simulink model "SpatialKineticsOffline"  (R2013a)
settings: Solver=ode4  StartTime=0.0  StopTime=tf  FixedStep=.001  RelTol=1e-3
PreLoadFcn:
  | load DarkLowerCoeffs
  | load DarkMiddleCoeffs
  | load DarkUpperCoeffs
  | load breaks
values from neighbouring files (symbols this model uses):
  alpha = [ -2.61*pcm -0.53*pcm ]    [SpatialKineticsOpenSourceMain.m]
  breaks = DarkLowerBreaks    [SpatialKineticsOpenSourceMain.m]
  BRIO = 4.266e7    (= 42660000)    [SpatialKineticsOpenSourceMain.m]
  cpc = 2414    [SpatialKineticsOpenSourceMain.m]
  cpp = 2414    [SpatialKineticsOpenSourceMain.m]
  DarkLowerCoeffs = ppDarkLower.coefs    [SpatialKineticsOpenSourceMain.m]
  DarkMiddleCoeffs = ppDarkMiddle.coefs    [SpatialKineticsOpenSourceMain.m]
  DarkRodWorthInserted = -5*Beta    (= -0.00815)    [SpatialKineticsOpenSourceMain.m]
  DarkUpperCoeffs = ppDarkUpper.coefs    [SpatialKineticsOpenSourceMain.m]
  downcomerTimeConstant = 5    [SpatialKineticsOpenSourceMain.m]
  downIO = 216.6*ones(1,3)    [SpatialKineticsOpenSourceMain.m]
  Kc1 = 1/(rho_secondary*V_secondary)    (= 0.00032726218348)    [SpatialKineticsOpenSourceMain.m]
  Kc2 = (h_secondary*A)/(cps*rho_secondary*V_secondary)    (= 1.23242359038)    [SpatialKineticsOpenSourceMain.m]
  Kh1 = 1/(rho_primary*V_primary)    (= 0.000447917898441)    [SpatialKineticsOpenSourceMain.m]
  Kh2 = (h_primary*A)/(cpp*rho_primary*V_primary)    (= 1.29038206968)    [SpatialKineticsOpenSourceMain.m]
  Kw1 = h_primary    (= 23800)    [SpatialKineticsOpenSourceMain.m]
  Kw2 = h_secondary    (= 24500)    [SpatialKineticsOpenSourceMain.m]
  Kw3 = A/(rho_tube*cpw*V_tube)    (= 0.000122049789882)    [SpatialKineticsOpenSourceMain.m]
  PHX_IO = [649.8 637.9 643.7]    [SpatialKineticsOpenSourceMain.m]
  PHX_PI_IO = 271.8    [SpatialKineticsOpenSourceMain.m]
  rate_pct = rate/100    [SpatialKineticsOfflineMain.m]
  rcp_activatetime = 20    [SpatialKineticsOpenSourceMain.m]
  rcpt = 0.1    [SpatialKineticsOpenSourceMain.m]
  reactor_PI_IO = 0.8574    [SpatialKineticsOpenSourceMain.m]
  SVIO = zeros(1,17)    [SpatialKineticsOpenSourceMain.m]
  Ts = 0.001    [SpatialKineticsOpenSourceMain.m]
  xfc0 = -Atemp\btemp*u0    [SpatialKineticsOpenSourceMain.m]
  zone1_IO = [1.041 0.01764 0.04848]    [SpatialKineticsOpenSourceMain.m]
  zone1_thermal_IO = [1044 658.3]    [SpatialKineticsOpenSourceMain.m]
  zone2_IO = [1.098 0.0186 0.05114]    [SpatialKineticsOpenSourceMain.m]
  zone2_thermal_IO = [1083 675.9]    [SpatialKineticsOpenSourceMain.m]
  zone3_IO = [0.9147 0.01549 0.04259]    [SpatialKineticsOpenSourceMain.m]
  zone3_thermal_IO = [1031 692.5]    [SpatialKineticsOpenSourceMain.m]
libraries: simulink x36
(part 5 of 5)

== system SpatialKineticsOffline/RX #4/Neutron Kinetics and Thermal Hydraulics/Temperature Reactivity Feedback2 ==
  In1 : Inport
  Sum : Sum  Inputs=|+-
  reactivity feedback matrix : Gain  Gain=alpha  Multiplication=Matrix(K*u)
  reactivity reference temperature : Constant  Value=xfc0  VectorParams1D=off
  Out1 : Outport
  wires:
  reactivity reference temperature/1 -> Sum/2
  Sum/1 -> reactivity feedback matrix/1
  reactivity feedback matrix/1 -> Out1/1
  In1/1 -> Sum/1

== system SpatialKineticsOffline/RX #4/Neutron Kinetics and Thermal Hydraulics/Temperature Reactivity Feedback3 ==
  In1 : Inport
  Sum : Sum  Inputs=|+-
  reactivity feedback matrix : Gain  Gain=alpha  Multiplication=Matrix(K*u)
  reactivity reference temperature : Constant  Value=xfc0  VectorParams1D=off
  Out1 : Outport
  wires:
  reactivity reference temperature/1 -> Sum/2
  Sum/1 -> reactivity feedback matrix/1
  reactivity feedback matrix/1 -> Out1/1
  In1/1 -> Sum/1

== matlab function SpatialKineticsOffline/RX #1/Neutron Kinetics and Thermal Hydraulics/Reactor Thermal-Hydraulics Zone 1/MATLAB Function ==
  data: m_dot input; Q_rx input; constants input; y output; T_c input; x input; x_dot output
function [y,x_dot] =FuelCoolantHX(m_dot,Q_rx,constants,T_c,x)

%The differential equations herein describe the lumped thermal-hydraulics
%of the fuel-coolant system.

cpc=constants(1);
cpf=constants(2);
mc=constants(3);
mf=constants(4);
uh=constants(5);
Ar=constants(6);

A=[-(uh*Ar)/(mf*cpf), (uh*Ar)/(mf*cpf); (uh*Ar)/(mc*cpc), -(uh*Ar)/(mc*cpc)-(2*m_dot)/mc];

K=125000000/3;

b=[K/(mf*cpf), 0; 0 2*m_dot/mc];

u=[Q_rx; T_c];

x_dot=A*x+b*u;

C=[1 0; 0 1; 0 2];
D=[0 0;0 0; 0 -1];

y=C*x+D*u;

return

== matlab function SpatialKineticsOffline/RX #2/Downcomer mixing dynamics/MATLAB Function1 ==
  data: m1 input; y output; mtotal output; m2 input; m3 input; t1 input; t2 input; t3 input; constants input; xdot output; x input
function [y,mtotal,xdot] = downcomermixingdynamics(m1,m2,m3,t1,t2,t3,constants,x)
%#codegen

mtotal = m1+m2+m3; %total mass flowrate

tau = constants(2); %plenum/downcomer effective time constant

A = [-1/tau 0 0;...
    0 -1/tau 0;...
    0 0 -1/tau];

B = [1/tau 0 0;...
    0 1/tau 0;...
    0 0 1/tau];

%Clear that the input is mass-flowrate weighted temperatures
u = [m1/mtotal * t1;...
    m2/mtotal * t2;...
    m3/mtotal * t3];

xdot = A*x + B*u;

y = [1 1 1]*x; %output is the linear combination of these states

return

== matlab function SpatialKineticsOffline/RX #1/Neutron Kinetics and Thermal Hydraulics/MATLAB Function ==
  data: DarkLowerCoeffs input; RodWorthLower output; DarkMiddleCoeffs input; DarkUpperCoeffs input; breaks input; RodWithdrawn input; RodWorthMiddle output; RodWorthUpper output
function [RodWorthLower,RodWorthMiddle,RodWorthUpper] = RodWorthIAEACurveFit(DarkLowerCoeffs,DarkMiddleCoeffs,DarkUpperCoeffs,breaks,...
    RodWithdrawn)

persistent L M U

for i = 1:length(breaks)-1
    if RodWithdrawn >= breaks(i) && RodWithdrawn < breaks(i+1)
        L = polyval(DarkLowerCoeffs(i,:),RodWithdrawn - breaks(i));
        M = polyval(DarkMiddleCoeffs(i,:),RodWithdrawn - breaks(i));
        U = polyval(DarkUpperCoeffs(i,:),RodWithdrawn - breaks(i));
        RodWorthLower = L;
        RodWorthMiddle = M;
        RodWorthUpper = U;
        return
    else
        L = 0;
        M = 0;
        U = 0;
        continue
    end
end

RodWorthLower = L;
RodWorthMiddle = M;
RodWorthUpper = U;

== matlab function SpatialKineticsOffline/RX #1/Neutron Kinetics and Thermal Hydraulics/Reactor Thermal-Hydraulics Zone 2/MATLAB Function ==
  data: m_dot input; Q_rx input; constants input; y output; T_c input; x input; x_dot output
function [y,x_dot] =FuelCoolantHX(m_dot,Q_rx,constants,T_c,x)

cpc=constants(1);
cpf=constants(2);
mc=constants(3);
mf=constants(4);
uh=constants(5);
Ar=constants(6);

A=[-(uh*Ar)/(mf*cpf), (uh*Ar)/(mf*cpf); (uh*Ar)/(mc*cpc), -(uh*Ar)/(mc*cpc)-(2*m_dot)/mc];

K=125000000/3;

b=[K/(mf*cpf), 0; 0 2*m_dot/mc];

u=[Q_rx; T_c];

x_dot=A*x+b*u;

C=[1 0; 0 1; 0 2];
D=[0 0;0 0; 0 -1];

y=C*x+D*u;

return

== matlab function SpatialKineticsOffline/RX #1/Neutron Kinetics and Thermal Hydraulics/Zone 3 Kinetics1 ==
  data: PROMPTN1 input; PROMPTN2 input; DELAYEDN1 input; DELAYEDN2 input; pkeparams input; rho_temp input; x input; y output; xdot output
function [y,xdot] = Zone3Kinetics(PROMPTN1,PROMPTN2,DELAYEDN1,DELAYEDN2,pkeparams,rho_temp,x)
%#codegen
% 
% %Unpackage the prompt and delayed neutron sources
% 
% %Prompt neuton unpackaging
N1 = PROMPTN1;
N2 = PROMPTN2;

% %Delayed neutron unpackaging
D1 = DELAYEDN1;
D2 = DELAYEDN2;

%PKE parameter load
Beta = pkeparams(1); B1 = pkeparams(2); B2 = pkeparams(3); 
L1 = pkeparams(8); L2 = pkeparams(9); 
lambda = pkeparams(14);

%Reactivity coupling effects from other zones
alpha = (1-Beta)/lambda;
%The numerical values (0.005 and 0.002) included herein represent the
%neutronic coupling coefficients that couple the delayed and prompt
%neutrons to other core regions.  It is quickly seen that these are
%translated into a reactivity.
rho_1 = lambda*0.002*(alpha*(N1/x(1))+0.002*(1/lambda)*D1/x(1));
rho_2 = lambda*0.005*(alpha*(N2/x(1))+0.005*(1/lambda)*D2/x(1));

% %Total reactivity

%Reactor Point Kinetics State Equation
rho_t=rho_temp+rho_1+rho_2;

A = [(rho_t-Beta)/lambda L1/lambda L2/lambda;...
    B1 -L1 0;...
    B2 0 -L2];

C = [1 0 0;...
    0 L1 L2];

xdot = zeros(3,1,'double');
xdot = A*x;
y = zeros(2,1,'double');
y = C*x;

return

== matlab function SpatialKineticsOffline/RX #2/Neutron Kinetics and Thermal Hydraulics1/MATLAB Function ==
  data: DarkLowerCoeffs input; RodWorthLower output; DarkMiddleCoeffs input; DarkUpperCoeffs input; breaks input; RodWithdrawn input; RodWorthMiddle output; RodWorthUpper output
function [RodWorthLower,RodWorthMiddle,RodWorthUpper] = RodWorthIAEACurveFit(DarkLowerCoeffs,DarkMiddleCoeffs,DarkUpperCoeffs,breaks,...
    RodWithdrawn)

persistent L M U

for i = 1:length(breaks)-1
    if RodWithdrawn >= breaks(i) && RodWithdrawn < breaks(i+1)
        L = polyval(DarkLowerCoeffs(i,:),RodWithdrawn - breaks(i));
        M = polyval(DarkMiddleCoeffs(i,:),RodWithdrawn - breaks(i));
        U = polyval(DarkUpperCoeffs(i,:),RodWithdrawn - breaks(i));
        RodWorthLower = L;
        RodWorthMiddle = M;
        RodWorthUpper = U;
        return
    else
        L = 0;
        M = 0;
        U = 0;
        continue
    end
end

RodWorthLower = L;
RodWorthMiddle = M;
RodWorthUpper = U;

== matlab function SpatialKineticsOffline/RX #2/Neutron Kinetics and Thermal Hydraulics1/Zone 2 Kinetics1 ==
  data: PROMPTN1 input; PROMPTN2 input; DELAYEDN1 input; DELAYEDN2 input; pkeparams input; rho_temp input; x input; y output; xdot output
function [y,xdot] = Zone2Kinetics(PROMPTN1,PROMPTN2,DELAYEDN1,DELAYEDN2,pkeparams,rho_temp,x)
%#codegen
% 
% K=reshape(Lcoupling,12,12); %Reshape the coupling matrix
% 
% %Unpackage the prompt and delayed neutron sources
% 
% %Prompt neuton unpackaging
N1 = PROMPTN1;
N2 = PROMPTN2;
% N2 = PROMPTN(2); N3 = PROMPTN(3); N4 = PROMPTN(4);
% N5 = PROMPTN(5); N6 = PROMPTN(6); N7 = PROMPTN(7);
% N8 = PROMPTN(8); N9 = PROMPTN(9); N10 = PROMPTN(10);
% N11 = PROMPTN(11); N12 = PROMPTN(12);
% 
% %Delayed neutron unpackaging
D1 = DELAYEDN1;
D2 = DELAYEDN2;
% D2 = DELAYEDN(2); D3 = DELAYEDN(3); D4 = DELAYEDN(4);
% D5 = DELAYEDN(5); D6 = DELAYEDN(6); D7 = DELAYEDN(7);
% D8 = DELAYEDN(8); D9 = DELAYEDN(9); D10 = DELAYEDN(10);
% D11 = DELAYEDN(11); D12 = DELAYEDN(12);

%PKE parameter load
Beta = pkeparams(1); B1 = pkeparams(2); B2 = pkeparams(3); B3 = pkeparams(4);
B4 = pkeparams(5); B5 = pkeparams(6); B6 = pkeparams(7); L1 = pkeparams(8);
L2 = pkeparams(9); L3 = pkeparams(10); L4 = pkeparams(11); L5 = pkeparams(12);
L6 = pkeparams(13); lambda = pkeparams(14);

%Reactivity coupling effects from other zones
alpha = (1-Beta)/lambda;
% 
rho_1 = lambda*0.005*(alpha*(N1/x(1))+0.005*(1/lambda)*D1/x(1));
rho_2 = lambda*0.005*(alpha*(N2/x(1))+0.005*(1/lambda)*D2/x(1));
% rho_3 = lambda*K(11,3)*(alpha*(N3/x(1))+(1/lambda)*D3/x(1));
% rho_4 = lambda*K(11,4)*(alpha*(N4/x(1))+(1/lambda)*D4/x(1));
% rho_5 = lambda*K(11,5)*(alpha*(N5/x(1))+(1/lambda)*D5/x(1));
% rho_6 = lambda*K(11,6)*(alpha*(N6/x(1))+(1/lambda)*D6/x(1));
% rho_7 = lambda*K(11,7)*(alpha*(N7/x(1))+(1/lambda)*D7/x(1));
% rho_8 = lambda*K(11,8)*(alpha*(N8/x(1))+(1/lambda)*D8/x(1));
% rho_9 = lambda*K(11,9)*(alpha*(N9/x(1))+(1/lambda)*D9/x(1));
% rho_10 = lambda*K(11,10)*(alpha*(N10/x(1))+(1/lambda)*D10/x(1));
% % rho_11 = lambda*K(11,11)*(alpha*(N11/x(1))+(1/lambda)*D11/x(1));
% rho_12 = lambda*K(11,12)*(alpha*(N12/x(1))+(1/lambda)*D12/x(1));
% 
% %Total reactivity
% 
% rho_t=rho_temp+rho_1+rho_2+rho_3+rho_4+rho_5+rho_6+rho_7+rho_8+rho_9+rho_10+rho_12;

%Reactor Point Kinetics State Equation
rho_t=rho_temp+rho_1+rho_2;

A = [(rho_t-Beta)/lambda L1/lambda L2/lambda;...
    B1 -L1 0;...
    B2 0 -L2];

C = [1 0 0;...
    0 L1 L2];

xdot = zeros(3,1,'double');
xdot = A*x;
y = zeros(2,1,'double');
y = C*x;

return

== matlab function SpatialKineticsOffline/RX #4/Downcomer mixing dynamics/MATLAB Function1 ==
  data: m1 input; y output; mtotal output; m2 input; m3 input; t1 input; t2 input; t3 input; constants input; xdot output; x input
function [y,mtotal,xdot] = downcomermixingdynamics(m1,m2,m3,t1,t2,t3,constants,x)
%#codegen

mtotal = m1+m2+m3; %total mass flowrate

tau = constants(2); %plenum/downcomer effective time constant

A = [-1/tau 0 0;...
    0 -1/tau 0;...
    0 0 -1/tau];

B = [1/tau 0 0;...
    0 1/tau 0;...
    0 0 1/tau];

%Clear that the input is mass-flowrate weighted temperatures
u = [m1/mtotal * t1;...
    m2/mtotal * t2;...
    m3/mtotal * t3];

xdot = A*x + B*u;

y = [1 1 1]*x; %output is the linear combination of these states

return

== matlab function SpatialKineticsOffline/RX #1/Primary Heat Exchanger Lumped Model #1/MATLAB Function ==
  data: x input; dx output; Thi_input input; Tci_input input; mdoth_input input; mdotc_input input; hxpar input
function dx  = fcn(x,Thi_input,Tci_input,mdoth_input,mdotc_input,hxpar)
%#codegen

%%%%% Temperature inputs
Thi = Thi_input;
Tci = Tci_input;

%%%%% Mass flow rate inputs
mdoth = mdoth_input;
mdotc = mdotc_input;

%%%%%% Parameters
kh1 = hxpar(1);
kh2 = hxpar(2);
kc1 = hxpar(3);
kc2 = hxpar(4);
kw1   = hxpar(5);
kw2   = hxpar(6);
kw3   = hxpar(7);

%%%%% States
%%%%% x = [x1 x2 x3]^T
%%%%% x1 is the hot-leg inlet temp
%%%%% x2 is the cold-leg inlet temp
%%%%% x3 is the wall temp
x1 = x(1);
x2 = x(2);
x3 = x(3);

%%%%% State equation
dx1 = -kh2*(x1-x3) + kh1*mdoth*(Thi-x1);
dx2 = kc2*(x3-x2) + kc1*mdotc*(Tci-x2);
dx3 = kw3*kw1*(x1-x3) - kw3*kw2*(x3-x2);

dx  = [dx1;dx2;dx3];

% %%%%%  Heat Transfer Output in MegaWatts
% HXout = mdoth*cpp*(Thi-x1) * 1e-6; 
% 
% %%%%% outlet Temperatures
% Tho = x(1);
% Tco = x(2);

== matlab function SpatialKineticsOffline/RX #3/Neutron Kinetics and Thermal Hydraulics1/Reactor Thermal-Hydraulics Zone 3/MATLAB Function ==
  data: m_dot input; Q_rx input; constants input; y output; T_c input; x input; x_dot output
function [y,x_dot] =FuelCoolantHX(m_dot,Q_rx,constants,T_c,x)

cpc=constants(1);
cpf=constants(2);
mc=constants(3);
mf=constants(4);
uh=constants(5);
Ar=constants(6);

A=[-(uh*Ar)/(mf*cpf), (uh*Ar)/(mf*cpf); (uh*Ar)/(mc*cpc), -(uh*Ar)/(mc*cpc)-(2*m_dot)/mc];

K=125000000/3;

b=[K/(mf*cpf), 0; 0 2*m_dot/mc];

u=[Q_rx; T_c];

x_dot=A*x+b*u;

C=[1 0; 0 1; 0 2];
D=[0 0;0 0; 0 -1];

y=C*x+D*u;

return

== matlab function SpatialKineticsOffline/RX #3/Neutron Kinetics and Thermal Hydraulics1/Zone 3 Kinetics1 ==
  data: PROMPTN1 input; PROMPTN2 input; DELAYEDN1 input; DELAYEDN2 input; pkeparams input; rho_temp input; x input; y output; xdot output
function [y,xdot] = Zone3Kinetics(PROMPTN1,PROMPTN2,DELAYEDN1,DELAYEDN2,pkeparams,rho_temp,x)
%#codegen
% 
% K=reshape(Lcoupling,12,12); %Reshape the coupling matrix
% 
% %Unpackage the prompt and delayed neutron sources
% 
% %Prompt neuton unpackaging
N1 = PROMPTN1;
N2 = PROMPTN2;
% N2 = PROMPTN(2); N3 = PROMPTN(3); N4 = PROMPTN(4);
% N5 = PROMPTN(5); N6 = PROMPTN(6); N7 = PROMPTN(7);
% N8 = PROMPTN(8); N9 = PROMPTN(9); N10 = PROMPTN(10);
% N11 = PROMPTN(11); N12 = PROMPTN(12);
% 
% %Delayed neutron unpackaging
D1 = DELAYEDN1;
D2 = DELAYEDN2;
% D2 = DELAYEDN(2); D3 = DELAYEDN(3); D4 = DELAYEDN(4);
% D5 = DELAYEDN(5); D6 = DELAYEDN(6); D7 = DELAYEDN(7);
% D8 = DELAYEDN(8); D9 = DELAYEDN(9); D10 = DELAYEDN(10);
% D11 = DELAYEDN(11); D12 = DELAYEDN(12);

%PKE parameter load
Beta = pkeparams(1); B1 = pkeparams(2); B2 = pkeparams(3); B3 = pkeparams(4);
B4 = pkeparams(5); B5 = pkeparams(6); B6 = pkeparams(7); L1 = pkeparams(8);
L2 = pkeparams(9); L3 = pkeparams(10); L4 = pkeparams(11); L5 = pkeparams(12);
L6 = pkeparams(13); lambda = pkeparams(14);

%Reactivity coupling effects from other zones
alpha = (1-Beta)/lambda;
% 
rho_1 = lambda*0.002*(alpha*(N1/x(1))+0.002*(1/lambda)*D1/x(1));
rho_2 = lambda*0.005*(alpha*(N2/x(1))+0.005*(1/lambda)*D2/x(1));
% rho_3 = lambda*K(11,3)*(alpha*(N3/x(1))+(1/lambda)*D3/x(1));
% rho_4 = lambda*K(11,4)*(alpha*(N4/x(1))+(1/lambda)*D4/x(1));
% rho_5 = lambda*K(11,5)*(alpha*(N5/x(1))+(1/lambda)*D5/x(1));
% rho_6 = lambda*K(11,6)*(alpha*(N6/x(1))+(1/lambda)*D6/x(1));
% rho_7 = lambda*K(11,7)*(alpha*(N7/x(1))+(1/lambda)*D7/x(1));
% rho_8 = lambda*K(11,8)*(alpha*(N8/x(1))+(1/lambda)*D8/x(1));
% rho_9 = lambda*K(11,9)*(alpha*(N9/x(1))+(1/lambda)*D9/x(1));
% rho_10 = lambda*K(11,10)*(alpha*(N10/x(1))+(1/lambda)*D10/x(1));
% % rho_11 = lambda*K(11,11)*(alpha*(N11/x(1))+(1/lambda)*D11/x(1));
% rho_12 = lambda*K(11,12)*(alpha*(N12/x(1))+(1/lambda)*D12/x(1));
% 
% %Total reactivity
% 
% rho_t=rho_temp+rho_1+rho_2+rho_3+rho_4+rho_5+rho_6+rho_7+rho_8+rho_9+rho_10+rho_12;

%Reactor Point Kinetics State Equation
rho_t=rho_temp+rho_1+rho_2;

A = [(rho_t-Beta)/lambda L1/lambda L2/lambda;...
    B1 -L1 0;...
    B2 0 -L2];

C = [1 0 0;...
    0 L1 L2];

xdot = zeros(3,1,'double');
xdot = A*x;
y = zeros(2,1,'double');
y = C*x;

return

== matlab function SpatialKineticsOffline/RX #2/Primary Heat Exchanger Lumped Model #4/MATLAB Function ==
  data: x input; dx output; Thi_input input; Tci_input input; mdoth_input input; mdotc_input input; hxpar input
function dx  = fcn(x,Thi_input,Tci_input,mdoth_input,mdotc_input,hxpar)
%#codegen

%%%%% Temperature inputs
Thi = Thi_input;
Tci = Tci_input;

%%%%% Mass flow rate inputs
mdoth = mdoth_input;
mdotc = mdotc_input;

%%%%%% Parameters
kh1 = hxpar(1);
kh2 = hxpar(2);
kc1 = hxpar(3);
kc2 = hxpar(4);
kw1   = hxpar(5);
kw2   = hxpar(6);
kw3   = hxpar(7);

%%%%% States
%%%%% x = [x1 x2 x3]^T
%%%%% x1 is the hot-leg inlet temp
%%%%% x2 is the cold-leg inlet temp
%%%%% x3 is the wall temp
x1 = x(1);
x2 = x(2);
x3 = x(3);

%%%%% State equation
dx1 = -kh2*(x1-x3) + kh1*mdoth*(Thi-x1);
dx2 = kc2*(x3-x2) + kc1*mdotc*(Tci-x2);
dx3 = kw3*kw1*(x1-x3) - kw3*kw2*(x3-x2);

dx  = [dx1;dx2;dx3];

% %%%%%  Heat Transfer Output in MegaWatts
% HXout = mdoth*cpp*(Thi-x1) * 1e-6; 
% 
% %%%%% outlet Temperatures
% Tho = x(1);
% Tco = x(2);

== matlab function SpatialKineticsOffline/RX #4/Neutron Kinetics and Thermal Hydraulics/Reactor Thermal-Hydraulics Zone 1/MATLAB Function ==
  data: m_dot input; Q_rx input; constants input; y output; T_c input; x input; x_dot output
function [y,x_dot] =FuelCoolantHX(m_dot,Q_rx,constants,T_c,x)

cpc=constants(1);
cpf=constants(2);
mc=constants(3);
mf=constants(4);
uh=constants(5);
Ar=constants(6);

A=[-(uh*Ar)/(mf*cpf), (uh*Ar)/(mf*cpf); (uh*Ar)/(mc*cpc), -(uh*Ar)/(mc*cpc)-(2*m_dot)/mc];

K=125000000/3;

b=[K/(mf*cpf), 0; 0 2*m_dot/mc];

u=[Q_rx; T_c];

x_dot=A*x+b*u;

C=[1 0; 0 1; 0 2];
D=[0 0;0 0; 0 -1];

y=C*x+D*u;

return

== matlab function SpatialKineticsOffline/RX #4/Neutron Kinetics and Thermal Hydraulics/Reactor Thermal-Hydraulics Zone 3/MATLAB Function ==
  data: m_dot input; Q_rx input; constants input; y output; T_c input; x input; x_dot output
function [y,x_dot] =FuelCoolantHX(m_dot,Q_rx,constants,T_c,x)

cpc=constants(1);
cpf=constants(2);
mc=constants(3);
mf=constants(4);
uh=constants(5);
Ar=constants(6);

A=[-(uh*Ar)/(mf*cpf), (uh*Ar)/(mf*cpf); (uh*Ar)/(mc*cpc), -(uh*Ar)/(mc*cpc)-(2*m_dot)/mc];

K=125000000/3;

b=[K/(mf*cpf), 0; 0 2*m_dot/mc];

u=[Q_rx; T_c];

x_dot=A*x+b*u;

C=[1 0; 0 1; 0 2];
D=[0 0;0 0; 0 -1];

y=C*x+D*u;

return

== matlab function SpatialKineticsOffline/RX #4/Neutron Kinetics and Thermal Hydraulics/Zone 3 Kinetics1 ==
  data: PROMPTN1 input; PROMPTN2 input; DELAYEDN1 input; DELAYEDN2 input; pkeparams input; rho_temp input; x input; y output; xdot output
function [y,xdot] = Zone3Kinetics(PROMPTN1,PROMPTN2,DELAYEDN1,DELAYEDN2,pkeparams,rho_temp,x)
%#codegen
% 
% K=reshape(Lcoupling,12,12); %Reshape the coupling matrix
% 
% %Unpackage the prompt and delayed neutron sources
% 
% %Prompt neuton unpackaging
N1 = PROMPTN1;
N2 = PROMPTN2;
% N2 = PROMPTN(2); N3 = PROMPTN(3); N4 = PROMPTN(4);
% N5 = PROMPTN(5); N6 = PROMPTN(6); N7 = PROMPTN(7);
% N8 = PROMPTN(8); N9 = PROMPTN(9); N10 = PROMPTN(10);
% N11 = PROMPTN(11); N12 = PROMPTN(12);
% 
% %Delayed neutron unpackaging
D1 = DELAYEDN1;
D2 = DELAYEDN2;
% D2 = DELAYEDN(2); D3 = DELAYEDN(3); D4 = DELAYEDN(4);
% D5 = DELAYEDN(5); D6 = DELAYEDN(6); D7 = DELAYEDN(7);
% D8 = DELAYEDN(8); D9 = DELAYEDN(9); D10 = DELAYEDN(10);
% D11 = DELAYEDN(11); D12 = DELAYEDN(12);

%PKE parameter load
Beta = pkeparams(1); B1 = pkeparams(2); B2 = pkeparams(3); B3 = pkeparams(4);
B4 = pkeparams(5); B5 = pkeparams(6); B6 = pkeparams(7); L1 = pkeparams(8);
L2 = pkeparams(9); L3 = pkeparams(10); L4 = pkeparams(11); L5 = pkeparams(12);
L6 = pkeparams(13); lambda = pkeparams(14);

%Reactivity coupling effects from other zones
alpha = (1-Beta)/lambda;
% 
rho_1 = lambda*0.002*(alpha*(N1/x(1))+0.002*(1/lambda)*D1/x(1));
rho_2 = lambda*0.005*(alpha*(N2/x(1))+0.005*(1/lambda)*D2/x(1));
% rho_3 = lambda*K(11,3)*(alpha*(N3/x(1))+(1/lambda)*D3/x(1));
% rho_4 = lambda*K(11,4)*(alpha*(N4/x(1))+(1/lambda)*D4/x(1));
% rho_5 = lambda*K(11,5)*(alpha*(N5/x(1))+(1/lambda)*D5/x(1));
% rho_6 = lambda*K(11,6)*(alpha*(N6/x(1))+(1/lambda)*D6/x(1));
% rho_7 = lambda*K(11,7)*(alpha*(N7/x(1))+(1/lambda)*D7/x(1));
% rho_8 = lambda*K(11,8)*(alpha*(N8/x(1))+(1/lambda)*D8/x(1));
% rho_9 = lambda*K(11,9)*(alpha*(N9/x(1))+(1/lambda)*D9/x(1));
% rho_10 = lambda*K(11,10)*(alpha*(N10/x(1))+(1/lambda)*D10/x(1));
% % rho_11 = lambda*K(11,11)*(alpha*(N11/x(1))+(1/lambda)*D11/x(1));
% rho_12 = lambda*K(11,12)*(alpha*(N12/x(1))+(1/lambda)*D12/x(1));
% 
% %Total reactivity
% 
% rho_t=rho_temp+rho_1+rho_2+rho_3+rho_4+rho_5+rho_6+rho_7+rho_8+rho_9+rho_10+rho_12;

%Reactor Point Kinetics State Equation
rho_t=rho_temp+rho_1+rho_2;

A = [(rho_t-Beta)/lambda L1/lambda L2/lambda;...
    B1 -L1 0;...
    B2 0 -L2];

C = [1 0 0;...
    0 L1 L2];

xdot = zeros(3,1,'double');
xdot = A*x;
y = zeros(2,1,'double');
y = C*x;

return

== matlab function SpatialKineticsOffline/RX #3/Primary Heat Exchanger Lumped Model #4/MATLAB Function ==
  data: x input; dx output; Thi_input input; Tci_input input; mdoth_input input; mdotc_input input; hxpar input
function dx  = fcn(x,Thi_input,Tci_input,mdoth_input,mdotc_input,hxpar)
%#codegen

%%%%% Temperature inputs
Thi = Thi_input;
Tci = Tci_input;

%%%%% Mass flow rate inputs
mdoth = mdoth_input;
mdotc = mdotc_input;

%%%%%% Parameters
kh1 = hxpar(1);
kh2 = hxpar(2);
kc1 = hxpar(3);
kc2 = hxpar(4);
kw1   = hxpar(5);
kw2   = hxpar(6);
kw3   = hxpar(7);


%%%%% States
%%%%% x = [x1 x2 x3]^T
%%%%% x1 is the hot-leg inlet temp
%%%%% x2 is the cold-leg inlet temp
%%%%% x3 is the wall temp
x1 = x(1);
x2 = x(2);
x3 = x(3);

%%%%% State equation
dx1 = -kh2*(x1-x3) + kh1*mdoth*(Thi-x1);
dx2 = kc2*(x3-x2) + kc1*mdotc*(Tci-x2);
dx3 = kw3*kw1*(x1-x3) - kw3*kw2*(x3-x2);

dx  = [dx1;dx2;dx3];
% 
% %%%%%  Heat Transfer Output in MegaWatts
% HXout = mdoth*cpp*(Thi-x1) * 1e-6; 
% 
% %%%%% outlet Temperatures
% Tho = x(1);
% Tco = x(2);

== matlab function SpatialKineticsOffline/Brayton Cycle #3/MATLAB Function4 ==
  data: y output; Tturb_out output; Tcomp_out output; xdot output; Tcomp_in input; Tturb_in input; mdot input; constants input; x input
function [y,Tturb_out,Tcomp_out,xdot]=BraytonCycle(Tcomp_in,Tturb_in,mdot,constants,x)

eta_comp=constants(1); %compressor efficiency
eta_turb=constants(2); %turbine efficiency
r=constants(3); %isotropic pressure ratio
cpCO2_turb=constants(4); %specific heat capacity of gas (which is air)
cpCO2_comp=constants(5);
% rhoCO2=constants(6);
tau_turb=constants(7); %Compressor-turbine time constant

Tcomp_out=(Tcomp_in+273)*((r-1)/eta_comp+1)-273; %Compressor outlet temperature
Tturb_out=(Tturb_in+273)*(1-eta_turb*(1-(1/r)))-273; %Turbine outlet temperature

Pturb=mdot*cpCO2_turb*(Tturb_in-Tturb_out); %Turbine power
Pcomp=mdot*cpCO2_comp*(Tcomp_out-Tcomp_in); %Compressor power

u=Pturb-Pcomp; %Preliminary input to state space model;

%Our state is the mechanical / shaft power produced 

A=-1/tau_turb; 
B=1/tau_turb;
C=1;
D=0;

%We are calcuating only the net mechanical output power, for now.
xdot=A*x+B*u;
y=C*x+D*u;

return

== matlab function SpatialKineticsOffline/RX #4/Primary Heat Exchanger Lumped Model #4/MATLAB Function ==
  data: x input; dx output; Thi_input input; Tci_input input; mdoth_input input; mdotc_input input; hxpar input
function dx  = fcn(x,Thi_input,Tci_input,mdoth_input,mdotc_input,hxpar)
%#codegen

%%%%% Temperature inputs
Thi = Thi_input;
Tci = Tci_input;

%%%%% Mass flow rate inputs
mdoth = mdoth_input;
mdotc = mdotc_input;

%%%%%% Parameters
kh1 = hxpar(1);
kh2 = hxpar(2);
kc1 = hxpar(3);
kc2 = hxpar(4);
kw1   = hxpar(5);
kw2   = hxpar(6);
kw3   = hxpar(7);

%%%%% States
%%%%% x = [x1 x2 x3]^T
%%%%% x1 is the hot-leg inlet temp
%%%%% x2 is the cold-leg inlet temp
%%%%% x3 is the wall temp
x1 = x(1);
x2 = x(2);
x3 = x(3);

%%%%% State equation
dx1 = -kh2*(x1-x3) + kh1*mdoth*(Thi-x1);
dx2 = kc2*(x3-x2) + kc1*mdotc*(Tci-x2);
dx3 = kw3*kw1*(x1-x3) - kw3*kw2*(x3-x2);

dx  = [dx1;dx2;dx3];

% %%%%%  Heat Transfer Output in MegaWatts
% HXout = mdoth*cpp*(Thi-x1) * 1e-6; 
% 
% %%%%% outlet Temperatures
% Tho = x(1);
% Tco = x(2);

== matlab function SpatialKineticsOffline/RX #4/Primary Heat Exchanger Lumped Model #6/MATLAB Function ==
  data: x input; dx output; Thi_input input; Tci_input input; mdoth_input input; mdotc_input input; hxpar input
function dx  = fcn(x,Thi_input,Tci_input,mdoth_input,mdotc_input,hxpar)
%#codegen

%%%%% Temperature inputs
Thi = Thi_input;
Tci = Tci_input;

%%%%% Mass flow rate inputs
mdoth = mdoth_input;
mdotc = mdotc_input;

%%%%%% Parameters
kh1 = hxpar(1);
kh2 = hxpar(2);
kc1 = hxpar(3);
kc2 = hxpar(4);
kw1   = hxpar(5);
kw2   = hxpar(6);
kw3   = hxpar(7);

%%%%% States
%%%%% x = [x1 x2 x3]^T
%%%%% x1 is the hot-leg inlet temp
%%%%% x2 is the cold-leg inlet temp
%%%%% x3 is the wall temp
x1 = x(1);
x2 = x(2);
x3 = x(3);

%%%%% State equation
dx1 = -kh2*(x1-x3) + kh1*mdoth*(Thi-x1);
dx2 = kc2*(x3-x2) + kc1*mdotc*(Tci-x2);
dx3 = kw3*kw1*(x1-x3) - kw3*kw2*(x3-x2);

dx  = [dx1;dx2;dx3];

% %%%%%  Heat Transfer Output in MegaWatts
% HXout = mdoth*cpp*(Thi-x1) * 1e-6; 
% 
% %%%%% outlet Temperatures
% Tho = x(1);
% Tco = x(2);

== matlab function SpatialKineticsOffline/RX #3/Parasitic Heat Loss Resulting from DRACS HXs2/MATLAB Function ==
  data: T_hot input; P_MW output; T_cold input; mdoth input; cpp input; Ploss_MW output; Th_red output
function [P_MW, Ploss_MW,Th_red] = fcn(T_hot,T_cold,mdoth,cpp)
%#codegen

%%%%% Inputs
%%%%% T_hot is the hot-leg temperature from the reactor-thermal Hydraulics
%%%%% T_cold is the temperatue to the reactor-thermal hydraulics from the
%%%%% downcomer
%%%%% mdoth is the primary mass flow rate from the downcomer


% Power output
P = mdoth*cpp*(T_hot-T_cold);  % units [Watts]
P_MW = P * 1e-6;               % units[MegaWatts]

% 1% Parasitic heat loss
Ploss     = 0.01 * P;                   % units [Watts]
Ploss_MW = Ploss * 1e-6;               % units[MegaWatts]

% Hot leg reduction
Th_red = Ploss/mdoth/cpp;               % Hot-leg reduction

return

== matlab function SpatialKineticsOffline/RX #1/Parasitic Heat Loss Resulting from DRACS HXs/MATLAB Function ==
  data: T_hot input; P_MW output; T_cold input; mdoth input; cpp input; Ploss_MW output; Th_red output
function [P_MW, Ploss_MW,Th_red] = fcn(T_hot,T_cold,mdoth,cpp)
%#codegen

%%%%% Inputs
%%%%% T_hot is the hot-leg temperature from the reactor-thermal Hydraulics
%%%%% T_cold is the temperatue to the reactor-thermal hydraulics from the
%%%%% downcomer
%%%%% mdoth is the primary mass flow rate from the downcomer


% Power output
P = mdoth*cpp*(T_hot-T_cold);  % units [Watts]
P_MW = P * 1e-6;               % units[MegaWatts]

% 1% Parasitic heat loss
Ploss     = 0.01 * P;                   % units [Watts]
Ploss_MW = Ploss * 1e-6;               % units[MegaWatts]

% Hot leg reduction
Th_red = Ploss/mdoth/cpp;               % Hot-leg reduction

return
